simulink model "BThrottleError"  (R2024b)
settings: configuration reference "STM32H7_Config" (kept outside this file)
undefined symbols (not defined in the file): rThrottleDeltaError, tSystemsTask, VThrottleErrorHigh, VThrottleErrorLow
libraries: simulink x3
settings Model: DataDictionary=Master_Dictionary.sldd  EnableAccessToBaseWorkspace=off  Creator=torni  LastModifiedBy=Will
settings ConfigSetRef: SourceName=STM32H7_Config

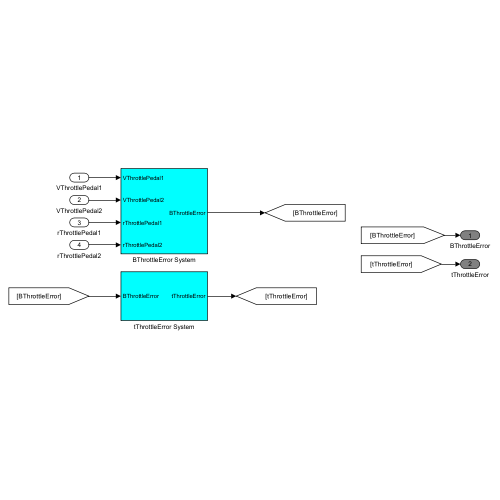
[thumbnail: Simulink's stored preview of the top-level diagram]
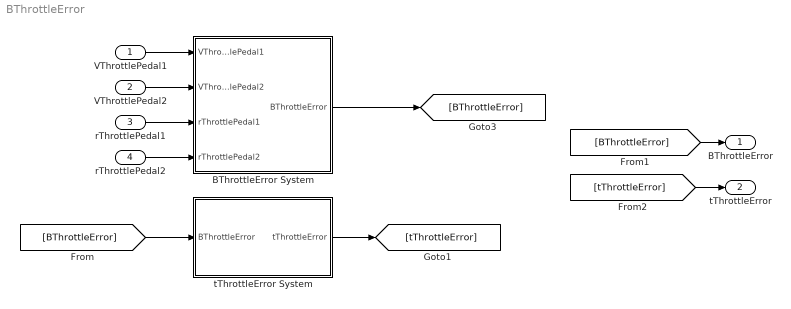
== system BThrottleError ==
  VThrottlePedal1 : Inport
  VThrottlePedal2 : Inport  Port=2
  rThrottlePedal1 : Inport  Port=3
  rThrottlePedal2 : Inport  Port=4
  BThrottleError System : Subsystem
  tThrottleError System : Subsystem
  BThrottleError : Outport  OutDataTypeStr=boolean  VectorParamsAs1DForOutWhenUnconnected=off
  tThrottleError : Outport  Port=2  OutDataTypeStr=double  VectorParamsAs1DForOutWhenUnconnected=off
  wires:
  VThrottlePedal1/1 -> BThrottleError System/1(VThrottlePedal1)
  VThrottlePedal2/1 -> BThrottleError System/2(VThrottlePedal2)
  rThrottlePedal1/1 -> BThrottleError System/3(rThrottlePedal1)
  rThrottlePedal2/1 -> BThrottleError System/4(rThrottlePedal2)
  BThrottleError System/1(BThrottleError) -> [BThrottleError]
  [BThrottleError] -> tThrottleError System/1(BThrottleError)
  [BThrottleError] -> BThrottleError/1
  tThrottleError System/1(tThrottleError) -> [tThrottleError]
  [tThrottleError] -> tThrottleError/1

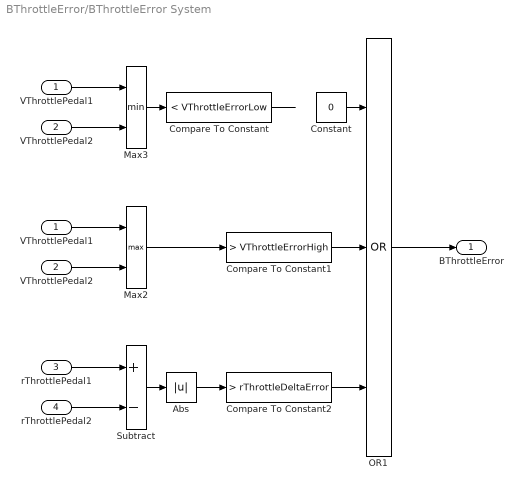
== system BThrottleError/BThrottleError System ==
  VThrottlePedal1 : Inport  OutDataTypeStr=double
  VThrottlePedal2 : Inport  Port=2  OutDataTypeStr=double
  rThrottlePedal1 : Inport  Port=3  OutDataTypeStr=double
  rThrottlePedal2 : Inport  Port=4  OutDataTypeStr=double
  Abs : Abs  SaturateOnIntegerOverflow=off
  Compare To Constant : simulink/Logic and Bit Operations/Compare To Constant  relop=<  const=VThrottleErrorLow  OutDataTypeStr=boolean
  Compare To Constant1 : simulink/Logic and Bit Operations/Compare To Constant  relop=>  const=VThrottleErrorHigh  OutDataTypeStr=boolean
  Compare To Constant2 : simulink/Logic and Bit Operations/Compare To Constant  relop=>  const=rThrottleDeltaError  OutDataTypeStr=boolean
  Constant : Constant  Value=0
  Max2 : MinMax  Function=max  Inputs=2
  Max3 : MinMax  Inputs=2
  OR1 : Logic  Operator=OR  Inputs=3  AllPortsSameDT=off  OutDataTypeStr=boolean
  Subtract : Sum  Inputs=+-
  "VThrottlePedal1 " : InportShadow  OutDataTypeStr=double
  "VThrottlePedal2 " : InportShadow  Port=2  OutDataTypeStr=double
  BThrottleError : Outport  OutDataTypeStr=boolean  VectorParamsAs1DForOutWhenUnconnected=off
  wires:
  Compare To Constant/1 -> ?
  rThrottlePedal2/1 -> Subtract/2
  rThrottlePedal1/1 -> Subtract/1
  Subtract/1 -> Abs/1
  Compare To Constant1/1 -> OR1/2
  Abs/1 -> Compare To Constant2/1
  VThrottlePedal2/1 -> Max2/2
  "VThrottlePedal2 "/1 -> Max3/2
  OR1/1 -> BThrottleError/1
  Max3/1 -> Compare To Constant/1
  Max2/1 -> Compare To Constant1/1
  Compare To Constant2/1 -> OR1/3
  VThrottlePedal1/1 -> Max2/1
  "VThrottlePedal1 "/1 -> Max3/1
  Constant/1 -> OR1/1

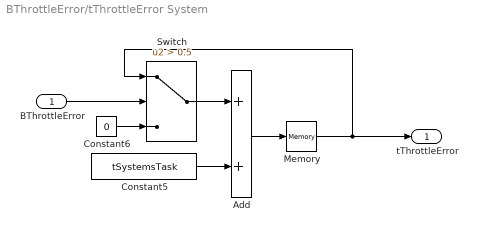
== system BThrottleError/tThrottleError System ==
  BThrottleError : Inport  OutDataTypeStr=boolean
  Add : Sum
  Constant5 : Constant  Value=tSystemsTask
  Constant6 : Constant  Value=0
  Memory : Memory  InheritSampleTime=on
  Switch : Switch  Criteria=u2 > Threshold  Threshold=0.5  SaturateOnIntegerOverflow=off  InputSameDT=off
  tThrottleError : Outport  OutDataTypeStr=double  VectorParamsAs1DForOutWhenUnconnected=off
  wires:
  Memory/1 -> tThrottleError/1, Switch/1
  Switch/1 -> Add/1
  Constant5/1 -> Add/2
  Add/1 -> Memory/1
  Constant6/1 -> Switch/3
  BThrottleError/1 -> Switch/2
